simulink library "asbhl20LGC"  (R2016b)
settings: Solver=VariableStepAuto  StartTime=0.0  StopTime=10.0  RelTol=1e-3
undefined symbols (not defined in the file): Tc
libraries: simulink x1
Description:
  | HL-20 landing gear control component module
settings Model: ExtModeAutoUpdateStatusClock=off  Creator=The MathWorks, Inc.  LastModifiedBy=The MathWorks, Inc.
settings DataIOCC: SaveFormat=Array  SignalLoggingSaveFormat=ModelDataLogs
settings OptimizationCC: BlockReduction=off  BooleanDataType=off
settings DebuggingCC: SaveWithParameterizedLinksMsg=none  UnderspecifiedInitializationDetection=Classic  MergeDetectMultiDrivingBlocksExec=none  SignalResolutionControl=TryResolveAllWithWarning  StrictBusMsg=Warning
settings HardwareCC: ProdBitPerPointer=32  ProdBitPerSizeT=32  ProdBitPerPtrDiffT=32  ProdLargestAtomicFloat=None  ProdIntDivRoundTo=Undefined  ProdEndianess=Unspecified  ProdWordSize=32  ProdHWDeviceType=32-bit Generic  TargetUnknown=on
settings ModelReferenceCC: PropagateSignalLabelsOutOfModel=off
settings ConfigComp: CovMetricSettings=dw  CovHtmlReporting=on  CovSaveCumulativeToWorkspaceVar=on  CovSaveSingleToWorkspaceVar=on  CovExternalEMLEnable=off

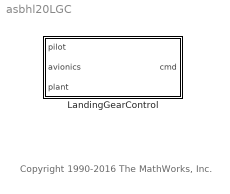
== system asbhl20LGC ==
  note: Copyright 1990-2016 The MathWorks, Inc.
  LandingGearControl : Subsystem  TreatAsAtomicUnit=on

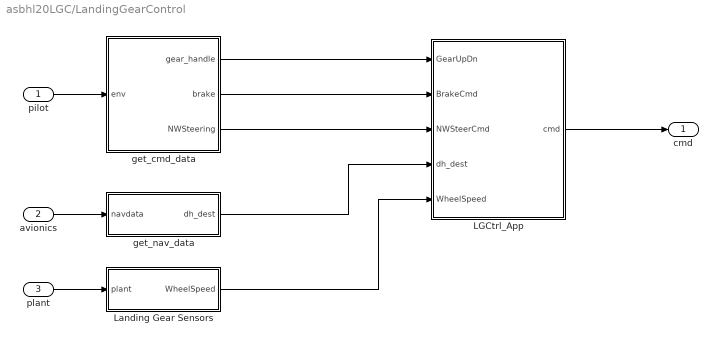
== system asbhl20LGC/LandingGearControl ==
  pilot : Inport
  avionics : Inport  Port=2
  plant : Inport  Port=3
  LGCtrl_App : Subsystem  TreatAsAtomicUnit=on  SystemSampleTime=Tc
  Landing Gear Sensors : Subsystem
  get_cmd_data : Subsystem
  get_nav_data : Subsystem
  " cmd" : Outport
  wires:
  pilot/1 -> get_cmd_data/1(env)
  LGCtrl_App/1(cmd) -> " cmd"/1
  get_cmd_data/1(gear_handle) -> LGCtrl_App/1(GearUpDn)
  get_cmd_data/2(brake) -> LGCtrl_App/2(BrakeCmd)
  get_cmd_data/3(NWSteering) -> LGCtrl_App/3(NWSteerCmd)
  plant/1 -> Landing Gear Sensors/1(plant)
  Landing Gear Sensors/1(WheelSpeed) -> LGCtrl_App/5(WheelSpeed)
  avionics/1 -> get_nav_data/1(navdata)
  get_nav_data/1(dh_dest) -> LGCtrl_App/4(dh_dest)

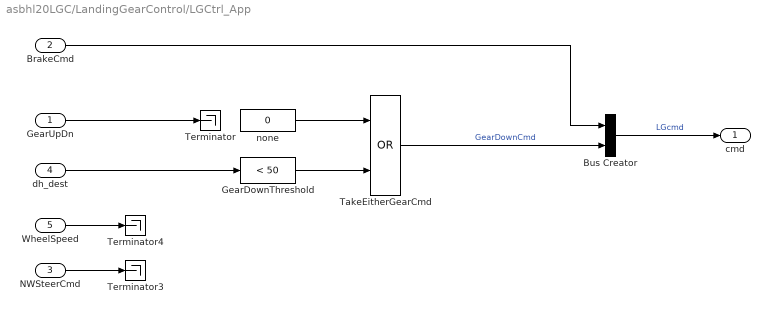
== system asbhl20LGC/LandingGearControl/LGCtrl_App ==
  GearUpDn : Inport
  BrakeCmd : Inport  Port=2
  NWSteerCmd : Inport  Port=3
  dh_dest : Inport  Port=4
  WheelSpeed : Inport  Port=5
  Bus Creator : BusCreator  Inputs=2
  GearDownThreshold : simulink/Logic and Bit Operations/Compare To Constant  relop=<  const=50  OutDataTypeStr=uint8  ZeroCross=off
  TakeEitherGearCmd : Logic  Operator=OR  IconShape=distinctive  AllPortsSameDT=off  OutDataTypeStr=boolean
  Terminator : Terminator
  Terminator3 : Terminator
  Terminator4 : Terminator
  none : Constant  Value=0  OutDataTypeStr=boolean
  cmd : Outport
  wires:
  NWSteerCmd/1 -> Terminator3/1
  WheelSpeed/1 -> Terminator4/1
  Bus Creator/1 -> cmd/1  "LGcmd"
  dh_dest/1 -> GearDownThreshold/1
  GearDownThreshold/1 -> TakeEitherGearCmd/2
  BrakeCmd/1 -> Bus Creator/1
  TakeEitherGearCmd/1 -> Bus Creator/2  "GearDownCmd"
  GearUpDn/1 -> Terminator/1
  none/1 -> TakeEitherGearCmd/1

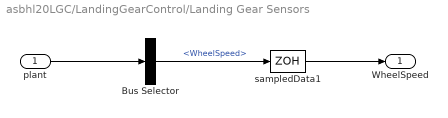
== system asbhl20LGC/LandingGearControl/Landing Gear Sensors ==
  plant : Inport
  Bus Selector : BusSelector  OutputSignals=LGData.WheelSpeed
  sampledData1 : ZeroOrderHold  SampleTime=Tc
  WheelSpeed : Outport
  wires:
  plant/1 -> Bus Selector/1
  Bus Selector/1 -> sampledData1/1  "<WheelSpeed>"
  sampledData1/1 -> WheelSpeed/1

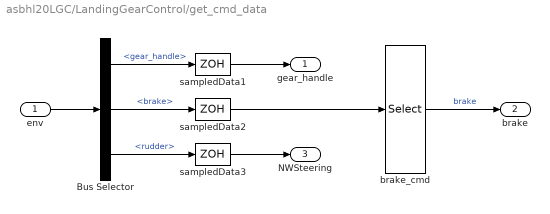
== system asbhl20LGC/LandingGearControl/get_cmd_data ==
  env : Inport
  Bus Selector : BusSelector  OutputSignals=gear_handle,brake,rudder
  brake_cmd : Selector  InputPortWidth=16  IndexOptions=Index vector (dialog)  Indices=1  OutputSizes=1
  sampledData1 : ZeroOrderHold  SampleTime=Tc
  sampledData2 : ZeroOrderHold  SampleTime=Tc
  sampledData3 : ZeroOrderHold  SampleTime=Tc
  gear_handle : Outport
  brake : Outport  Port=2
  NWSteering : Outport  Port=3
  wires:
  env/1 -> Bus Selector/1
  Bus Selector/2 -> sampledData2/1  "<brake>"
  Bus Selector/1 -> sampledData1/1  "<gear_handle>"
  Bus Selector/3 -> sampledData3/1  "<rudder>"
  brake_cmd/1 -> brake/1  "brake"
  sampledData2/1 -> brake_cmd/1
  sampledData1/1 -> gear_handle/1
  sampledData3/1 -> NWSteering/1

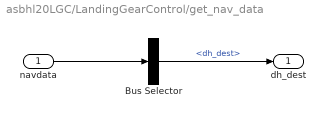
== system asbhl20LGC/LandingGearControl/get_nav_data ==
  navdata : Inport
  Bus Selector : BusSelector  OutputSignals=NavData.dh_dest
  dh_dest : Outport
  wires:
  navdata/1 -> Bus Selector/1
  Bus Selector/1 -> dh_dest/1  "<dh_dest>"
